simulink model "impedtest"  (Simulink 8.5)
settings: Solver=ode45  SolverMode=SingleTasking  StartTime=0.0  StopTime=1.0  RelTol=1e-3  AbsTol=1e-6
libraries: elements x32
settings Model: Creator=PC  LastModifiedBy=PC  ExtModeTrigMode=oneshot  ExtModeArmWhenConnect=off
settings DataIOCC: LimitDataPoints=off
settings OptimizationCC: BlockReduction=off  BooleanDataType=off  ExpressionDepthLimit=128
settings DebuggingCC: SaveWithParameterizedLinksMsg=none  SignalResolutionControl=TryResolveAllWithWarning  MultiTaskDSMMsg=warning  MultiTaskCondExecSysMsg=none  FcnCallInpInsideContextMsg=EnableAllAsError  StateNameClashWarn=none
settings HardwareCC: TargetUnknown=on

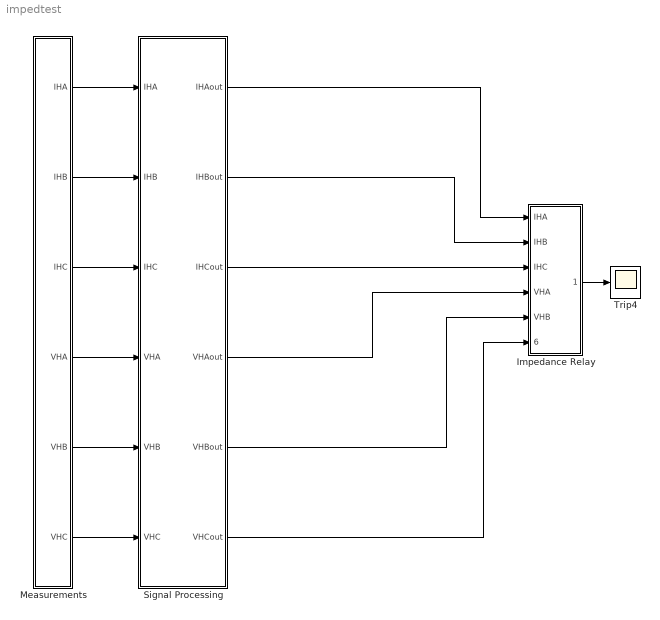
== system impedtest ==
  Impedance Relay : Subsystem  mask(Six-element Three-zone Impedance Relay){r=[0 0; -60 0; -65 -65; 0 -60], z2=[0 -0.5 ;1 0; 2 40; -0.5 0], z1=[0 -0.5 ;0.6 0; 1 21; -0.5 0]}
      mask prompts: r "Backward Zone Setting"; z2 "Zone 2 Setting"; z1 "Zone 1 Setting"
      mask help: Six-element three-zone (two forward and one backward) impedance relays for the backup protection of the high voltage winding.
  Measurements : Subsystem
  Signal Processing : Subsystem  mask(Signal Processing){ctx=31.5, cth=1.38, vs=13.8e3, vp=315e3, vector=11}
      mask prompts: ctx "CT Ratio of Low Voltage Side"; cth "CT Ratio of High Voltage Side"; vs "Secondary Voltage"; vp "Primary Voltage"; vector "Transformer Connection Vector"
      mask help: Transform analog measurements to digital format, including filtering, sampling . . .
  Trip4 : Scope
      settings: YMin=-1  YMax=1
  wires:
  Measurements/1(IHA) -> Signal Processing/1(IHA)
  Measurements/2(IHB) -> Signal Processing/2(IHB)
  Measurements/3(IHC) -> Signal Processing/3(IHC)
  Measurements/4(VHA) -> Signal Processing/4(VHA)
  Measurements/5(VHB) -> Signal Processing/5(VHB)
  Measurements/6(VHC) -> Signal Processing/6(VHC)
  Impedance Relay/1(Trip4) -> Trip4/1
  Signal Processing/1(IHAout) -> Impedance Relay/1(IHA)
  Signal Processing/2(IHBout) -> Impedance Relay/2(IHB)
  Signal Processing/3(IHCout) -> Impedance Relay/3(IHC)
  Signal Processing/4(VHAout) -> Impedance Relay/4(VHA)
  Signal Processing/5(VHBout) -> Impedance Relay/5(VHB)
  Signal Processing/6(VHCout) -> Impedance Relay/6(VHC)

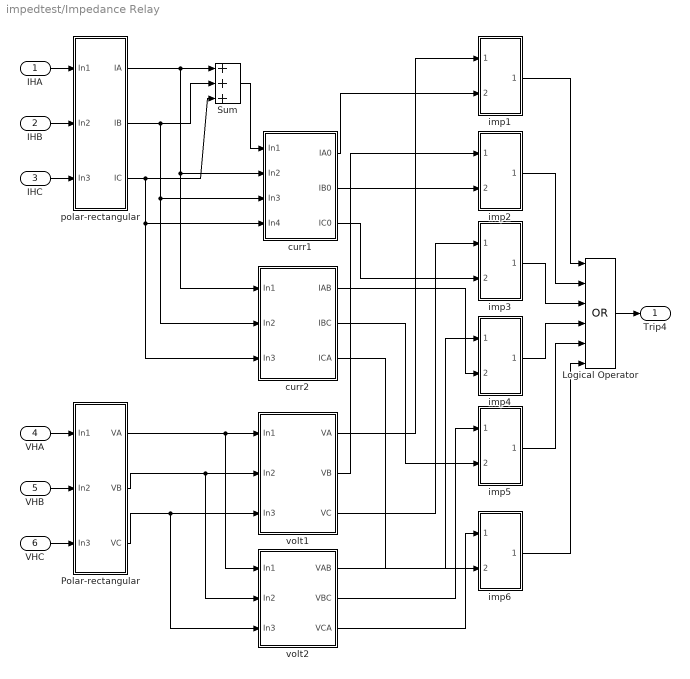
== system impedtest/Impedance Relay ==
  IHA : Inport
  IHB : Inport  Port=2
  IHC : Inport  Port=3
  VHA : Inport  Port=4
  VHB : Inport  Port=5
  VHC : Inport  Port=6
  " curr1" : Subsystem
  Logical Operator : Logic  Operator=OR  Inputs=6
  Polar-rectangular : Subsystem
  Sum : Sum  Inputs=+++  SaturateOnIntegerOverflow=on  InputSameDT=on  OutDataTypeStr=Inherit: Same as first input
  curr2 : Subsystem
  imp1 : Subsystem
  imp2 : Subsystem
  imp3 : Subsystem
  imp4 : Subsystem
  imp5 : Subsystem
  imp6 : Subsystem
  polar-rectangular : Subsystem
  volt1 : Subsystem
  volt2 : Subsystem
  Trip4 : Outport
  wires:
  " curr1"/1(IA0) -> imp1/2(In2)
  polar-rectangular/1(IA) -> Sum/1, " curr1"/2(In2), curr2/1(In1)
  volt1/1(VA) -> imp1/1(In1)
  Polar-rectangular/1(VA) -> volt1/1(In1), volt2/1(In1)
  Polar-rectangular/2(VB) -> volt1/2(In2), volt2/2(In2)
  polar-rectangular/2(IB) -> Sum/2, " curr1"/3(In3), curr2/2(In2)
  polar-rectangular/3(IC) -> Sum/3, " curr1"/4(In4), curr2/3(In3)
  Polar-rectangular/3(VC) -> volt1/3(In3), volt2/3(In3)
  Sum/1 -> " curr1"/1(In1)
  imp1/1(e1trip) -> Logical Operator/1
  imp2/1(e2trip) -> Logical Operator/2
  imp3/1(e3trip) -> Logical Operator/3
  imp4/1(e4trip) -> Logical Operator/4
  imp5/1(e5trip) -> Logical Operator/5
  imp6/1(e6trip) -> Logical Operator/6
  Logical Operator/1 -> Trip4/1
  " curr1"/2(IB0) -> imp2/2(In2)
  volt1/2(VB) -> imp2/1(In1)
  volt1/3(VC) -> imp3/1(In1)
  " curr1"/3(IC0) -> imp3/2(In2)
  volt2/1(VAB) -> imp4/1(In1)
  curr2/1(IAB) -> imp4/2(In2)
  volt2/2(VBC) -> imp5/1(In1)
  curr2/2(IBC) -> imp5/2(In2)
  volt2/3(VCA) -> imp6/1(In1)
  curr2/3(ICA) -> imp6/2(In2)
  IHA/1 -> polar-rectangular/1(In1)
  IHB/1 -> polar-rectangular/2(In2)
  IHC/1 -> polar-rectangular/3(In3)
  VHA/1 -> Polar-rectangular/1(In1)
  VHB/1 -> Polar-rectangular/2(In2)
  VHC/1 -> Polar-rectangular/3(In3)

== system impedtest/Measurements ==
  IHAf : FromFile  FileName=IHA2.mat  SampleTime=0
  IHBf : FromFile  FileName=IHB2.mat  SampleTime=0
  IHCf : FromFile  FileName=IHC2.mat  SampleTime=0
  VHAf : FromFile  FileName=VHA2.mat  SampleTime=0
  VHBf : FromFile  FileName=VHB2.mat  SampleTime=0
  VHCf : FromFile  FileName=VHC2.mat  SampleTime=0
  IHA : Outport
  IHB : Outport  Port=2
  IHC : Outport  Port=3
  VHA : Outport  Port=4
  VHB : Outport  Port=5
  VHC : Outport  Port=6
  wires:
  IHAf/1 -> IHA/1
  IHBf/1 -> IHB/1
  IHCf/1 -> IHC/1
  VHAf/1 -> VHA/1
  VHBf/1 -> VHB/1
  VHCf/1 -> VHC/1

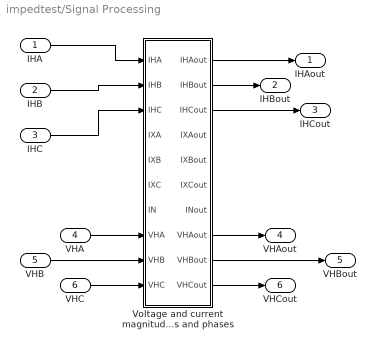
== system impedtest/Signal Processing ==
  IHA : Inport
  IHB : Inport  Port=2
  IHC : Inport  Port=3
  VHA : Inport  Port=4
  VHB : Inport  Port=5
  VHC : Inport  Port=6
  Voltage and current magnitudes and phases : Subsystem
  IHAout : Outport
  IHBout : Outport  Port=2
  IHCout : Outport  Port=3
  VHAout : Outport  Port=4
  VHBout : Outport  Port=5
  VHCout : Outport  Port=6
  wires:
  IHA/1 -> Voltage and current magnitudes and phases/1(IHA)
  IHB/1 -> Voltage and current magnitudes and phases/2(IHB)
  IHC/1 -> Voltage and current magnitudes and phases/3(IHC)
  Voltage and current magnitudes and phases/1(IHAout) -> IHAout/1
  Voltage and current magnitudes and phases/2(IHBout) -> IHBout/1
  Voltage and current magnitudes and phases/3(IHCout) -> IHCout/1
  Voltage and current magnitudes and phases/8(VHAout) -> VHAout/1
  Voltage and current magnitudes and phases/9(VHBout) -> VHBout/1
  Voltage and current magnitudes and phases/10(VHCout) -> VHCout/1
  VHA/1 -> Voltage and current magnitudes and phases/8(VHA)
  VHB/1 -> Voltage and current magnitudes and phases/9(VHB)
  VHC/1 -> Voltage and current magnitudes and phases/10(VHC)

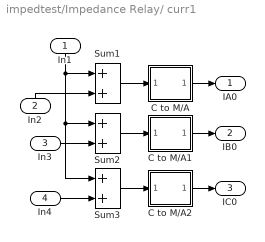
== system impedtest/Impedance Relay/ curr1 ==
  In1 : Inport
  In2 : Inport  Port=2
  In3 : Inport  Port=3
  In4 : Inport  Port=4
  C to M/A : Subsystem
  C to M/A1 : Subsystem
  C to M/A2 : Subsystem
  Sum1 : Sum  Inputs=2  SaturateOnIntegerOverflow=on  InputSameDT=on  OutDataTypeStr=Inherit: Same as first input
  Sum2 : Sum  Inputs=2  SaturateOnIntegerOverflow=on  InputSameDT=on  OutDataTypeStr=Inherit: Same as first input
  Sum3 : Sum  Inputs=2  SaturateOnIntegerOverflow=on  InputSameDT=on  OutDataTypeStr=Inherit: Same as first input
  IA0 : Outport
  IB0 : Outport  Port=2
  IC0 : Outport  Port=3
  wires:
  In1/1 -> Sum1/1, Sum2/1, Sum3/1
  Sum1/1 -> C to M/A/1(In1)
  In3/1 -> Sum2/2
  In2/1 -> Sum1/2
  Sum2/1 -> C to M/A1/1(In1)
  Sum3/1 -> C to M/A2/1(In1)
  In4/1 -> Sum3/2
  C to M/A/1(Out1) -> IA0/1
  C to M/A1/1(Out1) -> IB0/1
  C to M/A2/1(Out1) -> IC0/1

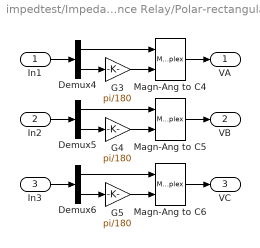
== system impedtest/Impedance Relay/Polar-rectangular ==
  In1 : Inport
  In2 : Inport  Port=2
  In3 : Inport  Port=3
  Demux4 : Demux  Outputs=2
  Demux5 : Demux  Outputs=2
  Demux6 : Demux  Outputs=2
  G3 : Gain  Gain=pi/180  SaturateOnIntegerOverflow=on  OutDataTypeStr=Inherit: Same as input  ParamDataTypeStr=Inherit: Same as input
  G4 : Gain  Gain=pi/180  SaturateOnIntegerOverflow=on  OutDataTypeStr=Inherit: Same as input  ParamDataTypeStr=Inherit: Same as input
  G5 : Gain  Gain=pi/180  SaturateOnIntegerOverflow=on  OutDataTypeStr=Inherit: Same as input  ParamDataTypeStr=Inherit: Same as input
  Magn-Ang to C4 : MagnitudeAngleToComplex
  Magn-Ang to C5 : MagnitudeAngleToComplex
  Magn-Ang to C6 : MagnitudeAngleToComplex
  VA : Outport
  VB : Outport  Port=2
  VC : Outport  Port=3
  wires:
  Demux4/1 -> Magn-Ang to C4/1
  Demux4/2 -> G3/1
  G3/1 -> Magn-Ang to C4/2
  Demux5/2 -> G4/1
  G4/1 -> Magn-Ang to C5/2
  Demux5/1 -> Magn-Ang to C5/1
  Demux6/2 -> G5/1
  G5/1 -> Magn-Ang to C6/2
  Demux6/1 -> Magn-Ang to C6/1
  Magn-Ang to C4/1 -> VA/1
  In1/1 -> Demux4/1
  Magn-Ang to C5/1 -> VB/1
  In2/1 -> Demux5/1
  Magn-Ang to C6/1 -> VC/1
  In3/1 -> Demux6/1

== system impedtest/Impedance Relay/curr2 ==
  In1 : Inport
  In2 : Inport  Port=2
  In3 : Inport  Port=3
  C to M/A : Subsystem
  C to M/A1 : Subsystem
  C to M/A2 : Subsystem
  Sum4 : Sum  Inputs=+-  SaturateOnIntegerOverflow=on  InputSameDT=on  OutDataTypeStr=Inherit: Same as first input
  Sum6 : Sum  Inputs=+-  SaturateOnIntegerOverflow=on  InputSameDT=on  OutDataTypeStr=Inherit: Same as first input
  Sum7 : Sum  Inputs=+-  SaturateOnIntegerOverflow=on  InputSameDT=on  OutDataTypeStr=Inherit: Same as first input
  IAB : Outport
  IBC : Outport  Port=2
  ICA : Outport  Port=3
  wires:
  In2/1 -> Sum4/2, Sum6/1
  In3/1 -> Sum6/2, Sum7/1
  In1/1 -> Sum4/1, Sum7/2
  Sum4/1 -> C to M/A/1(In1)
  C to M/A/1(Out1) -> IAB/1
  Sum6/1 -> C to M/A1/1(In1)
  C to M/A1/1(Out1) -> IBC/1
  Sum7/1 -> C to M/A2/1(In1)
  C to M/A2/1(Out1) -> ICA/1

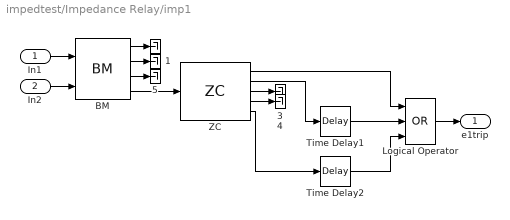
== system impedtest/Impedance Relay/imp1 ==
  In1 : Inport
  In2 : Inport  Port=2
   {,1,3..5} (5 alike) : Terminator
  BM : elements/BM  tpostv=none  plenv=4  tposti=none  pleni=4  tposts=none  plens=4  tpostz=none  plenz=4
  Logical Operator : Logic  Operator=OR  Inputs=3
  Time Delay1 : TransportDelay  DelayTime=0.2  BufferSize=2048
  Time Delay2 : TransportDelay  DelayTime=0.5  BufferSize=4096
  "ZC   " : elements/ZC     typez=Free expression  z1=z1  z2=z2  z3="[0  0; 0 0; 0 0; 0 0]"  z4="[0  0; 0 0; 0 0; 0 0]"  zr=r  fs=32*60
  e1trip : Outport
  wires:
  "ZC   "/2 -> Time Delay1/1
  "ZC   "/5 -> Time Delay2/1
  "ZC   "/3 -> " 3"/1
  "ZC   "/4 -> " 4"/1
  Time Delay1/1 -> Logical Operator/2
  Time Delay2/1 -> Logical Operator/3
  Logical Operator/1 -> e1trip/1
  BM/1 -> " "/1
  BM/2 -> " 1"/1
  BM/3 -> " 5"/1
  In1/1 -> BM/1
  In2/1 -> BM/2
  BM/4 -> "ZC   "/1
  "ZC   "/1 -> Logical Operator/1

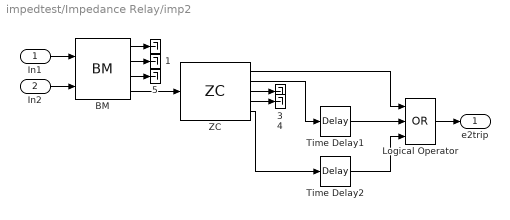
== system impedtest/Impedance Relay/imp2 ==
  In1 : Inport
  In2 : Inport  Port=2
   {,1,3..5} (5 alike) : Terminator
  BM : elements/BM  tpostv=none  plenv=4  tposti=none  pleni=4  tposts=none  plens=4  tpostz=none  plenz=4
  Logical Operator : Logic  Operator=OR  Inputs=3
  Time Delay1 : TransportDelay  DelayTime=0.2  BufferSize=2048
  Time Delay2 : TransportDelay  DelayTime=0.5  BufferSize=4096
  "ZC   " : elements/ZC     typez=Free expression  z1=z1  z2=z2  z3="[0  0; 0 0; 0 0; 0 0]"  z4="[0  0; 0 0; 0 0; 0 0]"  zr=r  fs=32*60
  e2trip : Outport
  wires:
  "ZC   "/1 -> Logical Operator/1
  BM/4 -> "ZC   "/1
  In2/1 -> BM/2
  In1/1 -> BM/1
  BM/3 -> " 5"/1
  BM/2 -> " 1"/1
  BM/1 -> " "/1
  Logical Operator/1 -> e2trip/1
  Time Delay2/1 -> Logical Operator/3
  Time Delay1/1 -> Logical Operator/2
  "ZC   "/4 -> " 4"/1
  "ZC   "/3 -> " 3"/1
  "ZC   "/5 -> Time Delay2/1
  "ZC   "/2 -> Time Delay1/1

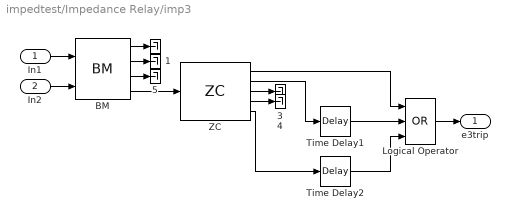
== system impedtest/Impedance Relay/imp3 ==
  In1 : Inport
  In2 : Inport  Port=2
   {,1,3..5} (5 alike) : Terminator
  BM : elements/BM  tpostv=none  plenv=4  tposti=none  pleni=4  tposts=none  plens=4  tpostz=none  plenz=4
  Logical Operator : Logic  Operator=OR  Inputs=3
  Time Delay1 : TransportDelay  DelayTime=0.2  BufferSize=2048
  Time Delay2 : TransportDelay  DelayTime=0.5  BufferSize=4096
  "ZC   " : elements/ZC     typez=Free expression  z1=z1  z2=z2  z3="[0  0; 0 0; 0 0; 0 0]"  z4="[0  0; 0 0; 0 0; 0 0]"  zr=r  fs=32*60
  e3trip : Outport
  wires:
  "ZC   "/2 -> Time Delay1/1
  "ZC   "/5 -> Time Delay2/1
  "ZC   "/3 -> " 3"/1
  "ZC   "/4 -> " 4"/1
  Time Delay1/1 -> Logical Operator/2
  Time Delay2/1 -> Logical Operator/3
  Logical Operator/1 -> e3trip/1
  BM/1 -> " "/1
  BM/2 -> " 1"/1
  BM/3 -> " 5"/1
  In1/1 -> BM/1
  In2/1 -> BM/2
  BM/4 -> "ZC   "/1
  "ZC   "/1 -> Logical Operator/1

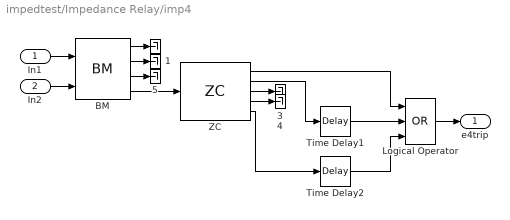
== system impedtest/Impedance Relay/imp4 ==
  In1 : Inport
  In2 : Inport  Port=2
   {,1,3..5} (5 alike) : Terminator
  BM : elements/BM  tpostv=none  plenv=4  tposti=none  pleni=4  tposts=none  plens=4  tpostz=none  plenz=4
  Logical Operator : Logic  Operator=OR  Inputs=3
  Time Delay1 : TransportDelay  DelayTime=0.2  BufferSize=2048
  Time Delay2 : TransportDelay  DelayTime=0.5  BufferSize=4096
  "ZC   " : elements/ZC     typez=Free expression  z1=z1  z2=z2  z3="[0  0; 0 0; 0 0; 0 0]"  z4="[0  0; 0 0; 0 0; 0 0]"  zr=r  fs=32*60
  e4trip : Outport
  wires:
  "ZC   "/1 -> Logical Operator/1
  BM/4 -> "ZC   "/1
  In2/1 -> BM/2
  In1/1 -> BM/1
  BM/3 -> " 5"/1
  BM/2 -> " 1"/1
  BM/1 -> " "/1
  Logical Operator/1 -> e4trip/1
  Time Delay2/1 -> Logical Operator/3
  Time Delay1/1 -> Logical Operator/2
  "ZC   "/4 -> " 4"/1
  "ZC   "/3 -> " 3"/1
  "ZC   "/5 -> Time Delay2/1
  "ZC   "/2 -> Time Delay1/1

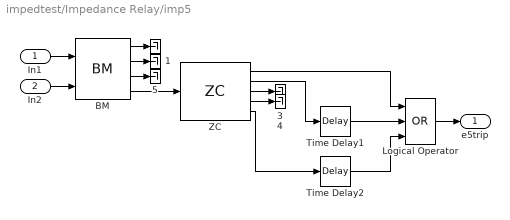
== system impedtest/Impedance Relay/imp5 ==
  In1 : Inport
  In2 : Inport  Port=2
   {,1,3..5} (5 alike) : Terminator
  BM : elements/BM  tpostv=none  plenv=4  tposti=none  pleni=4  tposts=none  plens=4  tpostz=none  plenz=4
  Logical Operator : Logic  Operator=OR  Inputs=3
  Time Delay1 : TransportDelay  DelayTime=0.2  BufferSize=2048
  Time Delay2 : TransportDelay  DelayTime=0.5  BufferSize=4096
  "ZC   " : elements/ZC     typez=Free expression  z1=z1  z2=z2  z3="[0  0; 0 0; 0 0; 0 0]"  z4="[0  0; 0 0; 0 0; 0 0]"  zr=r  fs=32*60
  e5trip : Outport
  wires:
  "ZC   "/2 -> Time Delay1/1
  "ZC   "/5 -> Time Delay2/1
  "ZC   "/3 -> " 3"/1
  "ZC   "/4 -> " 4"/1
  Time Delay1/1 -> Logical Operator/2
  Time Delay2/1 -> Logical Operator/3
  Logical Operator/1 -> e5trip/1
  BM/1 -> " "/1
  BM/2 -> " 1"/1
  BM/3 -> " 5"/1
  In1/1 -> BM/1
  In2/1 -> BM/2
  BM/4 -> "ZC   "/1
  "ZC   "/1 -> Logical Operator/1

== system impedtest/Impedance Relay/imp6 ==
  In1 : Inport
  In2 : Inport  Port=2
   {,1,3..5} (5 alike) : Terminator
  BM : elements/BM  tpostv=none  plenv=4  tposti=none  pleni=4  tposts=none  plens=4  tpostz=none  plenz=4
  Logical Operator : Logic  Operator=OR  Inputs=3
  Time Delay1 : TransportDelay  DelayTime=0.2  BufferSize=2048
  Time Delay2 : TransportDelay  DelayTime=0.5  BufferSize=4096
  "ZC   " : elements/ZC     typez=Free expression  z1=z1  z2=z2  z3="[0  0; 0 0; 0 0; 0 0]"  z4="[0  0; 0 0; 0 0; 0 0]"  zr=r  fs=32*60
  e6trip : Outport
  wires:
  "ZC   "/1 -> Logical Operator/1
  BM/4 -> "ZC   "/1
  In2/1 -> BM/2
  In1/1 -> BM/1
  BM/3 -> " 5"/1
  BM/2 -> " 1"/1
  BM/1 -> " "/1
  Logical Operator/1 -> e6trip/1
  Time Delay2/1 -> Logical Operator/3
  Time Delay1/1 -> Logical Operator/2
  "ZC   "/4 -> " 4"/1
  "ZC   "/3 -> " 3"/1
  "ZC   "/5 -> Time Delay2/1
  "ZC   "/2 -> Time Delay1/1

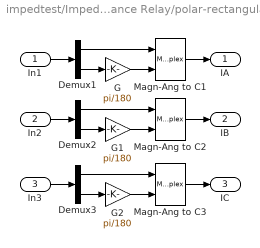
== system impedtest/Impedance Relay/polar-rectangular ==
  In1 : Inport
  In2 : Inport  Port=2
  In3 : Inport  Port=3
  Demux1 : Demux  Outputs=2
  Demux2 : Demux  Outputs=2
  Demux3 : Demux  Outputs=2
  G : Gain  Gain=pi/180  SaturateOnIntegerOverflow=on  OutDataTypeStr=Inherit: Same as input  ParamDataTypeStr=Inherit: Same as input
  G1 : Gain  Gain=pi/180  SaturateOnIntegerOverflow=on  OutDataTypeStr=Inherit: Same as input  ParamDataTypeStr=Inherit: Same as input
  G2 : Gain  Gain=pi/180  SaturateOnIntegerOverflow=on  OutDataTypeStr=Inherit: Same as input  ParamDataTypeStr=Inherit: Same as input
  Magn-Ang to C1 : MagnitudeAngleToComplex
  Magn-Ang to C2 : MagnitudeAngleToComplex
  Magn-Ang to C3 : MagnitudeAngleToComplex
  IA : Outport
  IB : Outport  Port=2
  IC : Outport  Port=3
  wires:
  Demux1/2 -> G/1
  G/1 -> Magn-Ang to C1/2
  Demux1/1 -> Magn-Ang to C1/1
  Demux2/2 -> G1/1
  G1/1 -> Magn-Ang to C2/2
  Demux2/1 -> Magn-Ang to C2/1
  Demux3/2 -> G2/1
  G2/1 -> Magn-Ang to C3/2
  Demux3/1 -> Magn-Ang to C3/1
  Magn-Ang to C1/1 -> IA/1
  In1/1 -> Demux1/1
  Magn-Ang to C2/1 -> IB/1
  In2/1 -> Demux2/1
  Magn-Ang to C3/1 -> IC/1
  In3/1 -> Demux3/1

== system impedtest/Impedance Relay/volt1 ==
  In1 : Inport
  In2 : Inport  Port=2
  In3 : Inport  Port=3
  C to M/A3 : Subsystem
  C to M/A4 : Subsystem
  C to M/A5 : Subsystem
  VA : Outport
  VB : Outport  Port=2
  VC : Outport  Port=3
  wires:
  In1/1 -> C to M/A3/1(In1)
  In2/1 -> C to M/A4/1(In1)
  In3/1 -> C to M/A5/1(In1)
  C to M/A3/1(Out1) -> VA/1
  C to M/A4/1(Out1) -> VB/1
  C to M/A5/1(Out1) -> VC/1

== system impedtest/Impedance Relay/volt2 ==
  In1 : Inport
  In2 : Inport  Port=2
  In3 : Inport  Port=3
  C to M/A6 : Subsystem
  C to M/A7 : Subsystem
  C to M/A8 : Subsystem
  Sum5 : Sum  Inputs=+-  SaturateOnIntegerOverflow=on  InputSameDT=on  OutDataTypeStr=Inherit: Same as first input
  Sum8 : Sum  Inputs=+-  SaturateOnIntegerOverflow=on  InputSameDT=on  OutDataTypeStr=Inherit: Same as first input
  Sum9 : Sum  Inputs=+-  SaturateOnIntegerOverflow=on  InputSameDT=on  OutDataTypeStr=Inherit: Same as first input
  VAB : Outport
  VBC : Outport  Port=2
  VCA : Outport  Port=3
  wires:
  In2/1 -> Sum5/2, Sum8/1
  In3/1 -> Sum8/2, Sum9/1
  In1/1 -> Sum5/1, Sum9/2
  Sum5/1 -> C to M/A6/1(In1)
  Sum8/1 -> C to M/A7/1(In1)
  Sum9/1 -> C to M/A8/1(In1)
  C to M/A6/1(Out1) -> VAB/1
  C to M/A7/1(Out1) -> VBC/1
  C to M/A8/1(Out1) -> VCA/1

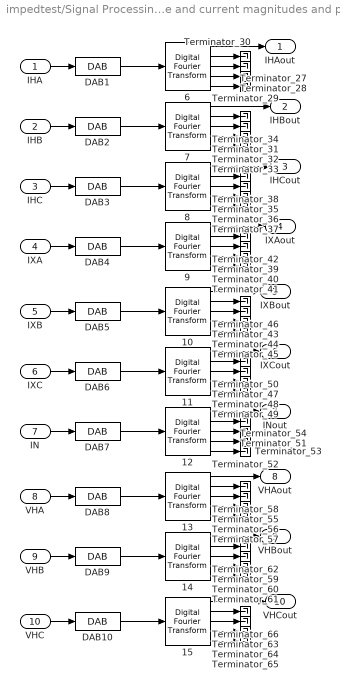
== system impedtest/Signal Processing/Voltage and current magnitudes and phases ==
  IHA : Inport
  IHB : Inport  Port=2
  IHC : Inport  Port=3
  IXA : Inport  Port=4
  IXB : Inport  Port=5
  IXC : Inport  Port=6
  IN : Inport  Port=7
  VHA : Inport  Port=8
  VHB : Inport  Port=9
  VHC : Inport  Port=10
   {6..15} (10 alike) : elements/   fo=60  window_size=32  harmonic=[1 2 3 4 5]
  DAB{1..10} (10 alike) : elements/DAB  filter=off  approx=Bessel  order=2  numerator=[]  denominator=[]  freq=360  resdis=off  vertres=12  xmax=10  winsize=32  G=1.0  fs=60*32
  Terminator_{27..66} (40 alike) : Terminator
  IHAout : Outport
  IHBout : Outport  Port=2
  IHCout : Outport  Port=3
  IXAout : Outport  Port=4
  IXBout : Outport  Port=5
  IXCout : Outport  Port=6
  INout : Outport  Port=7
  VHAout : Outport  Port=8
  VHBout : Outport  Port=9
  VHCout : Outport  Port=10
  wires:
  " 6"/2 -> Terminator_30/1
  " 6"/3 -> Terminator_27/1
  " 6"/4 -> Terminator_28/1
  " 6"/5 -> Terminator_29/1
  DAB1/1 -> " 6"/1
  IHA/1 -> DAB1/1
  " 7"/2 -> Terminator_34/1
  " 7"/3 -> Terminator_31/1
  " 7"/4 -> Terminator_32/1
  " 7"/5 -> Terminator_33/1
  DAB2/1 -> " 7"/1
  " 8"/2 -> Terminator_38/1
  " 8"/3 -> Terminator_35/1
  " 8"/4 -> Terminator_36/1
  " 8"/5 -> Terminator_37/1
  DAB3/1 -> " 8"/1
  " 9"/2 -> Terminator_42/1
  " 9"/3 -> Terminator_39/1
  " 9"/4 -> Terminator_40/1
  " 9"/5 -> Terminator_41/1
  DAB4/1 -> " 9"/1
  " 10"/2 -> Terminator_46/1
  " 10"/3 -> Terminator_43/1
  " 10"/4 -> Terminator_44/1
  " 10"/5 -> Terminator_45/1
  DAB5/1 -> " 10"/1
  " 11"/2 -> Terminator_50/1
  " 11"/3 -> Terminator_47/1
  " 11"/4 -> Terminator_48/1
  " 11"/5 -> Terminator_49/1
  DAB6/1 -> " 11"/1
  " 12"/2 -> Terminator_54/1
  " 12"/3 -> Terminator_51/1
  " 12"/4 -> Terminator_52/1
  " 12"/5 -> Terminator_53/1
  DAB7/1 -> " 12"/1
  " 13"/2 -> Terminator_58/1
  " 13"/3 -> Terminator_55/1
  " 13"/4 -> Terminator_56/1
  " 13"/5 -> Terminator_57/1
  DAB8/1 -> " 13"/1
  " 14"/2 -> Terminator_62/1
  " 14"/3 -> Terminator_59/1
  " 14"/4 -> Terminator_60/1
  " 14"/5 -> Terminator_61/1
  DAB9/1 -> " 14"/1
  " 15"/2 -> Terminator_66/1
  " 15"/3 -> Terminator_63/1
  " 15"/4 -> Terminator_64/1
  " 15"/5 -> Terminator_65/1
  DAB10/1 -> " 15"/1
  " 6"/1 -> IHAout/1
  " 7"/1 -> IHBout/1
  IHB/1 -> DAB2/1
  " 8"/1 -> IHCout/1
  IHC/1 -> DAB3/1
  " 9"/1 -> IXAout/1
  IXA/1 -> DAB4/1
  " 10"/1 -> IXBout/1
  IXB/1 -> DAB5/1
  " 11"/1 -> IXCout/1
  IXC/1 -> DAB6/1
  " 12"/1 -> INout/1
  IN/1 -> DAB7/1
  " 13"/1 -> VHAout/1
  VHA/1 -> DAB8/1
  " 14"/1 -> VHBout/1
  VHB/1 -> DAB9/1
  " 15"/1 -> VHCout/1
  VHC/1 -> DAB10/1

== system impedtest/Impedance Relay/ curr1/C to M/A ==
  In1 : Inport
  C to Magn-Ang : ComplexToMagnitudeAngle
  G : Gain  Gain=180/pi  SaturateOnIntegerOverflow=on  OutDataTypeStr=Inherit: Same as input  ParamDataTypeStr=Inherit: Same as input
  Mux1 : Mux  Inputs=2
  Out1 : Outport
  wires:
  C to Magn-Ang/2 -> G/1
  C to Magn-Ang/1 -> Mux1/1
  G/1 -> Mux1/2
  Mux1/1 -> Out1/1
  In1/1 -> C to Magn-Ang/1

== system impedtest/Impedance Relay/ curr1/C to M/A1 ==
  In1 : Inport
  C to Magn-Ang : ComplexToMagnitudeAngle
  G : Gain  Gain=180/pi  SaturateOnIntegerOverflow=on  OutDataTypeStr=Inherit: Same as input  ParamDataTypeStr=Inherit: Same as input
  Mux1 : Mux  Inputs=2
  Out1 : Outport
  wires:
  In1/1 -> C to Magn-Ang/1
  Mux1/1 -> Out1/1
  G/1 -> Mux1/2
  C to Magn-Ang/1 -> Mux1/1
  C to Magn-Ang/2 -> G/1

== system impedtest/Impedance Relay/ curr1/C to M/A2 ==
  In1 : Inport
  C to Magn-Ang : ComplexToMagnitudeAngle
  G : Gain  Gain=180/pi  SaturateOnIntegerOverflow=on  OutDataTypeStr=Inherit: Same as input  ParamDataTypeStr=Inherit: Same as input
  Mux1 : Mux  Inputs=2
  Out1 : Outport
  wires:
  C to Magn-Ang/2 -> G/1
  C to Magn-Ang/1 -> Mux1/1
  G/1 -> Mux1/2
  Mux1/1 -> Out1/1
  In1/1 -> C to Magn-Ang/1

== system impedtest/Impedance Relay/curr2/C to M/A ==
  In1 : Inport
  C to Magn-Ang : ComplexToMagnitudeAngle
  G : Gain  Gain=180/pi  SaturateOnIntegerOverflow=on  OutDataTypeStr=Inherit: Same as input  ParamDataTypeStr=Inherit: Same as input
  Mux1 : Mux  Inputs=2
  Out1 : Outport
  wires:
  C to Magn-Ang/2 -> G/1
  C to Magn-Ang/1 -> Mux1/1
  G/1 -> Mux1/2
  Mux1/1 -> Out1/1
  In1/1 -> C to Magn-Ang/1

== system impedtest/Impedance Relay/curr2/C to M/A1 ==
  In1 : Inport
  C to Magn-Ang : ComplexToMagnitudeAngle
  G : Gain  Gain=180/pi  SaturateOnIntegerOverflow=on  OutDataTypeStr=Inherit: Same as input  ParamDataTypeStr=Inherit: Same as input
  Mux1 : Mux  Inputs=2
  Out1 : Outport
  wires:
  In1/1 -> C to Magn-Ang/1
  Mux1/1 -> Out1/1
  G/1 -> Mux1/2
  C to Magn-Ang/1 -> Mux1/1
  C to Magn-Ang/2 -> G/1

== system impedtest/Impedance Relay/curr2/C to M/A2 ==
  In1 : Inport
  C to Magn-Ang : ComplexToMagnitudeAngle
  G : Gain  Gain=180/pi  SaturateOnIntegerOverflow=on  OutDataTypeStr=Inherit: Same as input  ParamDataTypeStr=Inherit: Same as input
  Mux1 : Mux  Inputs=2
  Out1 : Outport
  wires:
  C to Magn-Ang/2 -> G/1
  C to Magn-Ang/1 -> Mux1/1
  G/1 -> Mux1/2
  Mux1/1 -> Out1/1
  In1/1 -> C to Magn-Ang/1

== system impedtest/Impedance Relay/volt1/C to M/A3 ==
  In1 : Inport
  C to Magn-Ang : ComplexToMagnitudeAngle
  G : Gain  Gain=180/pi  SaturateOnIntegerOverflow=on  OutDataTypeStr=Inherit: Same as input  ParamDataTypeStr=Inherit: Same as input
  Mux1 : Mux  Inputs=2
  Out1 : Outport
  wires:
  In1/1 -> C to Magn-Ang/1
  Mux1/1 -> Out1/1
  G/1 -> Mux1/2
  C to Magn-Ang/1 -> Mux1/1
  C to Magn-Ang/2 -> G/1

== system impedtest/Impedance Relay/volt1/C to M/A4 ==
  In1 : Inport
  C to Magn-Ang : ComplexToMagnitudeAngle
  G : Gain  Gain=180/pi  SaturateOnIntegerOverflow=on  OutDataTypeStr=Inherit: Same as input  ParamDataTypeStr=Inherit: Same as input
  Mux1 : Mux  Inputs=2
  Out1 : Outport
  wires:
  C to Magn-Ang/2 -> G/1
  C to Magn-Ang/1 -> Mux1/1
  G/1 -> Mux1/2
  Mux1/1 -> Out1/1
  In1/1 -> C to Magn-Ang/1

== system impedtest/Impedance Relay/volt1/C to M/A5 ==
  In1 : Inport
  C to Magn-Ang : ComplexToMagnitudeAngle
  G : Gain  Gain=180/pi  SaturateOnIntegerOverflow=on  OutDataTypeStr=Inherit: Same as input  ParamDataTypeStr=Inherit: Same as input
  Mux1 : Mux  Inputs=2
  Out1 : Outport
  wires:
  In1/1 -> C to Magn-Ang/1
  Mux1/1 -> Out1/1
  G/1 -> Mux1/2
  C to Magn-Ang/1 -> Mux1/1
  C to Magn-Ang/2 -> G/1

== system impedtest/Impedance Relay/volt2/C to M/A6 ==
  In1 : Inport
  C to Magn-Ang : ComplexToMagnitudeAngle
  G : Gain  Gain=180/pi  SaturateOnIntegerOverflow=on  OutDataTypeStr=Inherit: Same as input  ParamDataTypeStr=Inherit: Same as input
  Mux1 : Mux  Inputs=2
  Out1 : Outport
  wires:
  C to Magn-Ang/2 -> G/1
  C to Magn-Ang/1 -> Mux1/1
  G/1 -> Mux1/2
  Mux1/1 -> Out1/1
  In1/1 -> C to Magn-Ang/1

== system impedtest/Impedance Relay/volt2/C to M/A7 ==
  In1 : Inport
  C to Magn-Ang : ComplexToMagnitudeAngle
  G : Gain  Gain=180/pi  SaturateOnIntegerOverflow=on  OutDataTypeStr=Inherit: Same as input  ParamDataTypeStr=Inherit: Same as input
  Mux1 : Mux  Inputs=2
  Out1 : Outport
  wires:
  In1/1 -> C to Magn-Ang/1
  Mux1/1 -> Out1/1
  G/1 -> Mux1/2
  C to Magn-Ang/1 -> Mux1/1
  C to Magn-Ang/2 -> G/1

== system impedtest/Impedance Relay/volt2/C to M/A8 ==
  In1 : Inport
  C to Magn-Ang : ComplexToMagnitudeAngle
  G : Gain  Gain=180/pi  SaturateOnIntegerOverflow=on  OutDataTypeStr=Inherit: Same as input  ParamDataTypeStr=Inherit: Same as input
  Mux1 : Mux  Inputs=2
  Out1 : Outport
  wires:
  C to Magn-Ang/2 -> G/1
  C to Magn-Ang/1 -> Mux1/1
  G/1 -> Mux1/2
  Mux1/1 -> Out1/1
  In1/1 -> C to Magn-Ang/1
